simulink model "mat_Lap_1_31"  (R2020b)
settings: Solver=VariableStepAuto  StartTime=0.0  StopTime=10  RelTol=1e-3
values from neighbouring files (symbols this model uses):
  x0 = X2(:,m)    [plot_lab9.m]
undefined symbols (not defined in the file or in its folder): b, c, d
libraries: simulink x1
settings Model: Creator=Maciek  LastModifiedBy=Maciek

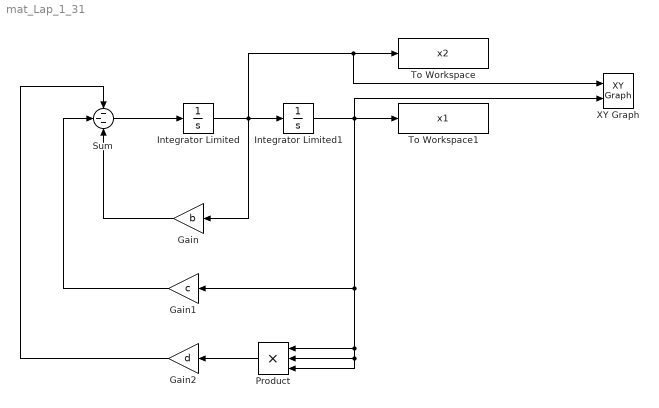
== system mat_Lap_1_31 ==
  Gain : Gain  Gain=b
  Gain1 : Gain  Gain=c
  Gain2 : Gain  Gain=d
  Integrator Limited : Integrator  InitialCondition=x0(1)  LimitOutput=on  UpperSaturationLimit=2  LowerSaturationLimit=-2
  Integrator Limited1 : Integrator  InitialCondition=x0(2)  LimitOutput=on  UpperSaturationLimit=2  LowerSaturationLimit=-2
  Product : Product  Inputs=3
  Sum : Sum  Inputs=---
  To Workspace : ToWorkspace  VariableName=x2  SampleTime=-1
      settings: Save2DSignal=2-D array (concatenate along first dimension)
  To Workspace1 : ToWorkspace  VariableName=x1  SampleTime=-1
      settings: Save2DSignal=2-D array (concatenate along first dimension)
  XY Graph : simulink/Sinks/XY Graph  xmin=-1  xmax=1  ymin=-1  ymax=1  st=-1
  wires:
  Sum/1 -> Integrator Limited/1
  Gain/1 -> Sum/3
  Gain1/1 -> Sum/2
  Gain2/1 -> Sum/1
  Product/1 -> Gain2/1
  Integrator Limited1/1 -> XY Graph/2, Gain1/1, Product/2, Product/3, Product/1, To Workspace1/1
  Integrator Limited/1 -> XY Graph/1, To Workspace/1, Gain/1, Integrator Limited1/1
